simulink model "TrustAI_ros"  (R2023b)
settings: Solver=FixedStepAuto  StartTime=0.0  StopTime=10.0  RelTol=1e-3
libraries: robotlib x3
settings Model: Creator=yuweiyang  LastModifiedBy=yuweiyang
settings OptimizationCC: EnhancedBackFolding=on  PassReuseOutputArgsAs=Individual arguments  ZeroExternalMemoryAtStartup=off  ZeroInternalMemoryAtStartup=off  MaxStackSize=64  OptimizeBlockOrder=speed  DifferentSizesBufferReuse=on  OptimizationCustomize=off  EfficientTunableParamExpr=on
settings DebuggingCC: ParameterTunabilityLossMsg=error
settings HardwareCC: ProdBitPerPointer=32  ProdBitPerSizeT=32  ProdBitPerPtrDiffT=32  ProdLargestAtomicFloat=None  ProdIntDivRoundTo=Undefined  ProdEndianess=Unspecified  ProdWordSize=32  ProdHWDeviceType=Generic->Unspecified (assume 32-bit Generic)
settings SFSimCC: MATLABDynamicMemAlloc=off
settings RTWCC: Description=Embedded Coder  SystemTargetFile=ert.tlc  HardwareBoard=Robot Operating System (ROS)  TLCOptions="-aInlineSetEventsForThisBaseRateFcn=TLC_FALSE -aSuppressMultiTaskScheduler=TLC_FALSE  -aRateBasedStepFcn=0"  GenCodeOnly=on  TemplateMakefile=ert_default_tmf  Toolchain=Catkin  TargetLang=C++
settings CodeAppCC: ForceParamTrailComments=on  IgnoreCustomStorageClasses=off  OperatorAnnotations=on  SimulinkDataObjDesc=on  SFDataObjDesc=on  InsertBlockDesc=on
settings ERTTargetCC: SupportContinuousTime=on

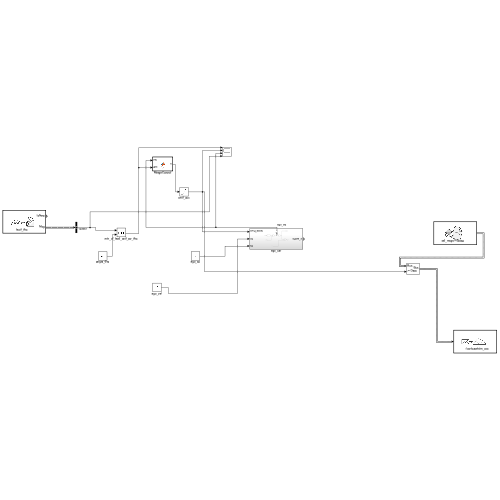
[thumbnail: Simulink's stored preview of the top-level diagram]
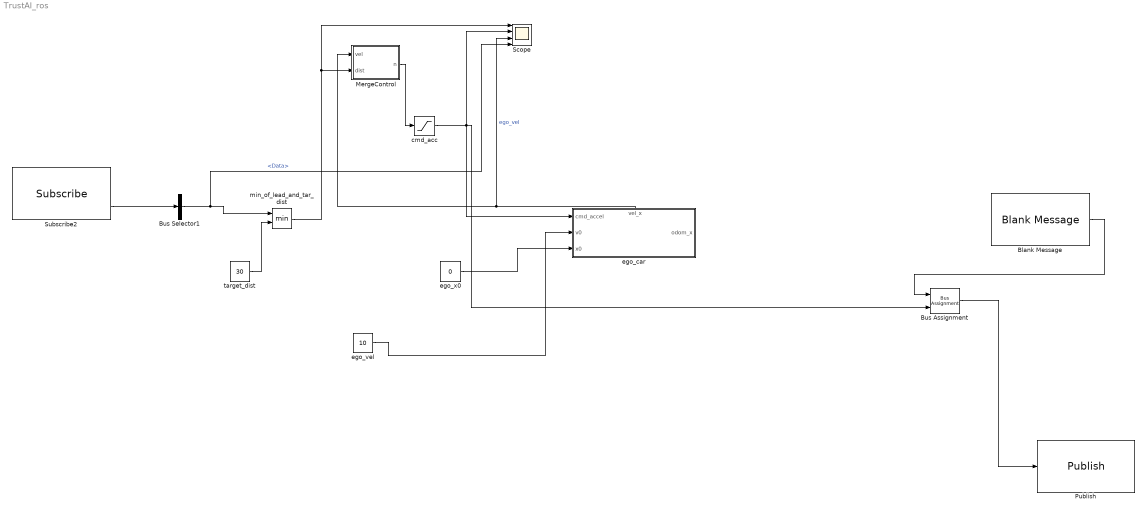
== system TrustAI_ros ==
  Blank Message : robotlib/Blank Message  messageClass=Message  entityType=std_msgs/Float64  messageType=std_msgs/Float64  SampleTime=inf  legacyBusStruct=off
  Bus Assignment : BusAssignment  AssignedSignals=Data
  Bus Selector1 : BusSelector  OutputSignals=Data
  MergeControl : MATLAB Function  TreatAsAtomicUnit=on
  Publish : robotlib/Publish  topicSource=Specify your own  topic=/car/state/sim_acc  messageType=std_msgs/Float64  legacyBusStruct=off  messageQueueLength=1
  Scope : Scope  NumInputPorts=4
  Subscribe2 : robotlib/Subscribe  topicSource=Specify your own  topic=lead_dist  messageType=std_msgs/Float64  SampleTime=-1  legacyBusStruct=off  messageQueueLength=1
  cmd_acc : Saturate  UpperLimit=3  LowerLimit=-1.5
  ego_car : Subsystem
      settings: PortSchema="{\"entries\":[{\"content\":{\"sides\":[{\"content\":{\"connectorIds\":[\"In1\",\"In2\",\"In3\"]},\"type\":\"ConnectorPlacement.EquallySpacedRectSide\",\"uuid\":\"81953a61-2087-4640-8924-dd2553d262e4\"},{\"content\":{\"connectorIds\":[\"Out1\"],\"side\":\"RIGHT\"},\"type\":\"ConnectorPlacement.EquallySpacedRectSide\",\"uuid\":\"3438fc64-880d-4339-a3b8-3c07203bfc0a\"},{\"content\":{\"connectorIds\":[\"Out2\"],\"side\":\"TOP\"},\"type\":\"ConnectorPlacement.EquallySpacedRectSide\",\"uuid\":\"5fb53f00-e2cd-4409-87c6-d9d884618a68\"}]},\"type\":\"ConnectorPlacement.EquallySpacedConnector\",\"uuid\":\"e0e50f07-b074-4548-b861-e4b426313971\"}],\"packageUris\":[\"http://schema.mathworks.com/mf0/Connector/R2020b\"],\"version\":\"1.0\"}"
  ego_vel : Constant  Value=10
  ego_x0 : Constant  Value=0
  min_of_lead_and_tar_dist : MinMax  Inputs=2
  target_dist : Constant  Value=30
  wires:
  target_dist/1 -> min_of_lead_and_tar_dist/2
  min_of_lead_and_tar_dist/1 -> Scope/1, MergeControl/2(dist)
  cmd_acc/1 -> Bus Assignment/2, ego_car/1(cmd_accel), Scope/2
  MergeControl/1(n) -> cmd_acc/1
  ego_x0/1 -> ego_car/3(x0)
  Bus Selector1/1 -> Scope/4, min_of_lead_and_tar_dist/1  "<Data>"
  ego_car/2(vel_x) -> Scope/3, MergeControl/1(vel)  "ego_vel"
  ego_vel/1 -> ego_car/2(v0)
  Subscribe2/2 -> Bus Selector1/1
  Bus Assignment/1 -> Publish/1
  Blank Message/1 -> Bus Assignment/1

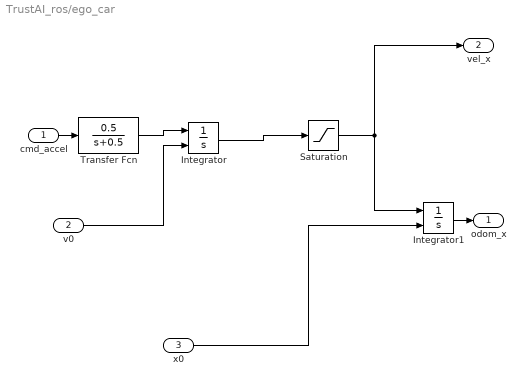
== system TrustAI_ros/ego_car ==
  cmd_accel : Inport
  v0 : Inport  Port=2
  x0 : Inport  Port=3
  Integrator : Integrator  InitialConditionSource=external
  Integrator1 : Integrator  InitialConditionSource=external
  Saturation : Saturate  UpperLimit=80  LowerLimit=0
  Transfer Fcn : TransferFcn  Numerator=[0.5]  Denominator=[1 0.5]
  odom_x : Outport
  vel_x : Outport  Port=2
  wires:
  v0/1 -> Integrator/2
  cmd_accel/1 -> Transfer Fcn/1
  Transfer Fcn/1 -> Integrator/1
  Integrator1/1 -> odom_x/1
  Integrator/1 -> Saturation/1
  x0/1 -> Integrator1/2
  Saturation/1 -> vel_x/1, Integrator1/1

== matlab function TrustAI_ros/MergeControl ==
  data: vel input; dist input; n output
function n  = fcn(vel, dist)
    k1 = 0.5;
    k2 = 0.1;
    headway = 5;
    vel_desire = 10;
    n = k1 * (dist - headway * vel) + k2 * (vel_desire - vel);
end
